simulink model "SVC_Modell_Changed"  (R2021a)
settings: Solver=ode1  StartTime=0.0  StopTime=t_Stop  FixedStep=0.1  RelTol=1e-3
values from neighbouring files (symbols this model uses):
  b_h = 0.5    [ParamterKamijiSVC_Changed.m]
  K_a = 0.1    [ParamterKamijiSVC_Changed.m]
  K_ac = 1.2    [ParamterKamijiSVC_Changed.m]
  K_vc = 6    [ParamterKamijiSVC_Changed.m]
  K_w = 0.9    [ParamterKamijiSVC_Changed.m]
  K_wc = 4    [ParamterKamijiSVC_Changed.m]
  n_h = 2    [ParamterKamijiSVC_Changed.m]
  P_kin = 1    [ParamterKamijiSVC_Changed.m]
  tau_a = 190    [ParamterKamijiSVC_Changed.m]
  tau_d = 7    [ParamterKamijiSVC_Changed.m]
  tau_LP = 0.1    [ParamterKamijiSVC_Changed.m]
undefined symbols (not defined in the file or in its folder): tau_MSI_unique
libraries: vrlib x3
settings Model: PauseTimes=1  Creator=BattiPerdator  LastModifiedBy=BattiPerdator

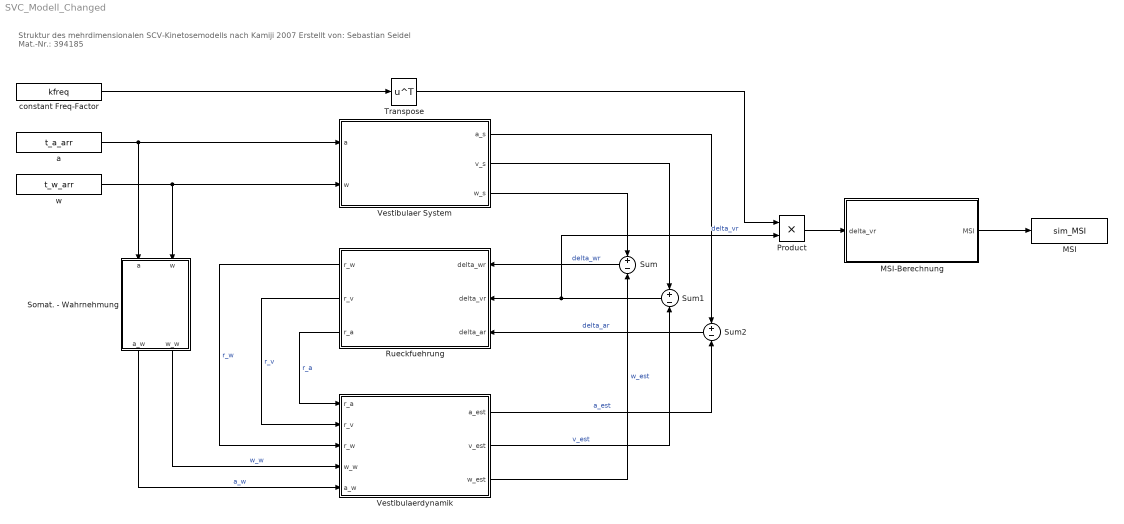
== system SVC_Modell_Changed ==
  note: Struktur des mehrdimensionalen SCV-Kinetosemodells nach Kamiji 2007
      | Erstellt von: Sebastian Seidel
      | Mat.-Nr.: 394185
  MSI : ToWorkspace  VariableName=sim_MSI  SampleTime=-1
  MSI-Berechnung : Subsystem
  Product : Product
  Rueckfuehrung : Subsystem
  Somat. - Wahrnehmung : Subsystem
  Sum : Sum  Inputs=+|-
  Sum1 : Sum  Inputs=+|-
  Sum2 : Sum  Inputs=+|-
  Transpose : Math  Operator=transpose  SaturateOnIntegerOverflow=on
  Vestibulaer System : Subsystem
  Vestibulaerdynamik : Subsystem
  "a " : FromWorkspace  VariableName=t_a_arr
  constant Freq-Factor : FromWorkspace  VariableName=kfreq
  w : FromWorkspace  VariableName=t_w_arr
  wires:
  w/1 -> Somat. - Wahrnehmung/2(w), Vestibulaer System/2(w)
  Somat. - Wahrnehmung/2(w_w) -> Vestibulaerdynamik/4(w_w)  "w_w"
  Somat. - Wahrnehmung/1(a_w) -> Vestibulaerdynamik/5(a_w)  "a_w"
  Vestibulaer System/1(a_s) -> Sum2/1
  Vestibulaer System/2(v_s) -> Sum1/1
  Vestibulaer System/3(w_s) -> Sum/1
  Vestibulaerdynamik/2(v_est) -> Sum1/2  "v_est"
  Rueckfuehrung/3(r_a) -> Vestibulaerdynamik/1(r_a)  "r_a"
  Rueckfuehrung/2(r_v) -> Vestibulaerdynamik/2(r_v)  "r_v"
  Rueckfuehrung/1(r_w) -> Vestibulaerdynamik/3(r_w)  "r_w"
  MSI-Berechnung/1(MSI) -> MSI/1
  Vestibulaerdynamik/1(a_est) -> Sum2/2  "a_est"
  Vestibulaerdynamik/3(w_est) -> Sum/2  "w_est"
  "a "/1 -> Somat. - Wahrnehmung/1(a), Vestibulaer System/1(a)
  Sum/1 -> Rueckfuehrung/1(delta_wr)  "delta_wr"
  Sum1/1 -> Product/2, Rueckfuehrung/2(delta_vr)  "delta_vr"
  Sum2/1 -> Rueckfuehrung/3(delta_ar)  "delta_ar"
  Product/1 -> MSI-Berechnung/1(delta_vr)
  constant Freq-Factor/1 -> Transpose/1
  Transpose/1 -> Product/1

== system SVC_Modell_Changed/MSI-Berechnung ==
  note: 0 ≤ MSI ≤ 1
  note: [-]
  note: [m/s²]
  delta_vr : Inport
  Hillfunktion : Subsystem
  Uebertragungsfunktion MSI : Subsystem
  MSI : Outport
  wires:
  delta_vr/1 -> Hillfunktion/1(delta_vr)
  Uebertragungsfunktion MSI/1(MSI) -> MSI/1
  Hillfunktion/1(h(delta_vr)) -> Uebertragungsfunktion MSI/1(h(delta_vr))

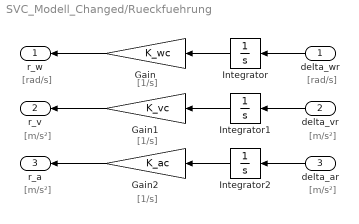
== system SVC_Modell_Changed/Rueckfuehrung ==
  note: [1/s]
  note: [rad/s]
  note: [m/s²]
  note: [m/s²]
  note: [rad/s]
  note: [m/s²]
  note: [m/s²]
  note: [1/s]
  note: [1/s]
  delta_wr : Inport
  delta_vr : Inport  Port=2
  delta_ar : Inport  Port=3
  Gain : Gain  Gain=K_wc
  Gain1 : Gain  Gain=K_vc
  Gain2 : Gain  Gain=K_ac
  Integrator : Integrator
  Integrator1 : Integrator
  Integrator2 : Integrator
  r_w : Outport
  r_v : Outport  Port=2
  r_a : Outport  Port=3
  wires:
  Gain/1 -> r_w/1
  Gain1/1 -> r_v/1
  Gain2/1 -> r_a/1
  delta_wr/1 -> Integrator/1
  Integrator/1 -> Gain/1
  delta_vr/1 -> Integrator1/1
  Integrator1/1 -> Gain1/1
  delta_ar/1 -> Integrator2/1
  Integrator2/1 -> Gain2/1

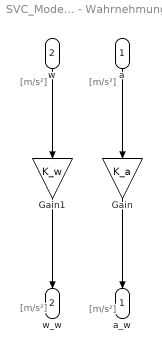
== system SVC_Modell_Changed/Somat. - Wahrnehmung ==
  note: [m/s²]
  note: [m/s²]
  note: [m/s²]
  note: [m/s²]
  a : Inport
  w : Inport  Port=2
  Gain : Gain  Gain=K_a
  Gain1 : Gain  Gain=K_w
  a_w : Outport
  w_w : Outport  Port=2
  wires:
  a/1 -> Gain/1
  Gain/1 -> a_w/1
  w/1 -> Gain1/1
  Gain1/1 -> w_w/1

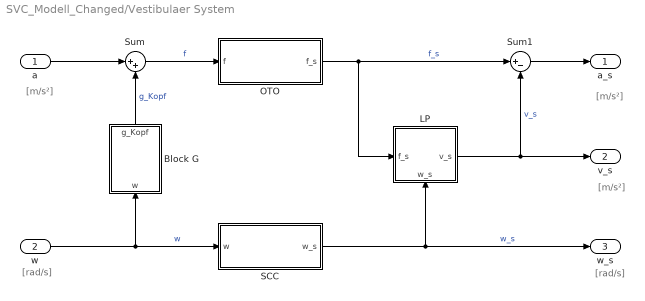
== system SVC_Modell_Changed/Vestibulaer System ==
  note: [m/s²]
  note: [m/s²]
  note: [m/s²]
  note: [rad/s]
  note: [rad/s]
  a : Inport
  w : Inport  Port=2
  Block G : Subsystem
  LP : Subsystem
      settings: PortSchema="{\"entries\":[{\"content\":{\"sides\":[{\"content\":{\"connectorIds\":[\"In1\"]},\"type\":\"ConnectorPlacement.EquallySpacedRectSide\",\"uuid\":\"fff2062c-4976-4e3f-90bd-2690d3961207\"},{\"content\":{\"connectorIds\":[\"Out1\"],\"side\":\"RIGHT\"},\"type\":\"ConnectorPlacement.EquallySpacedRectSide\",\"uuid\":\"f381f760-d607-432e-947a-7c2ed5cb0343\"},{\"content\":{\"connectorIds\":[],\"side\":\"TOP\"},\"type\":\"ConnectorPlacement.EquallySpacedRectSide\",\"uuid\":\"39b8ee05-57d9-4c64-9465-c67dc6896307\"},{\"content\":{\"connectorIds\":[\"In2\"],\"side\":\"BOTTOM\"},\"type\":\"ConnectorPlacement.EquallySpacedRectSide\",\"uuid\":\"95c95475-e280-41e4-b9b1-4b16bc0b77a9\"}]},\"type\":\"ConnectorPlacement.EquallySpacedConnector\",\"uuid\":\"1ef14ed4-54ab-4761-aaa8-a6dbdea02457\"}],\"packageUris\":[\"http://schema.mathworks.com/mf0/Connector/R2020b\"],\"version\":\"1.0\"}"
  OTO : Subsystem
  SCC : Subsystem
  Sum : Sum  Inputs=|++
  Sum1 : Sum  Inputs=|+-
  a_s : Outport
  v_s : Outport  Port=2
  w_s : Outport  Port=3
  wires:
  Block G/1(g_Kopf) -> Sum/2  "g_Kopf"
  a/1 -> Sum/1
  Sum/1 -> OTO/1(f)  "f"
  Sum1/1 -> a_s/1
  OTO/1(f_s) -> LP/1(f_s), Sum1/1  "f_s"
  LP/1(v_s) -> Sum1/2, v_s/1  "v_s"
  w/1 -> SCC/1(w), Block G/1(w)  "w"
  SCC/1(w_s) -> LP/2(w_s), w_s/1  "w_s"

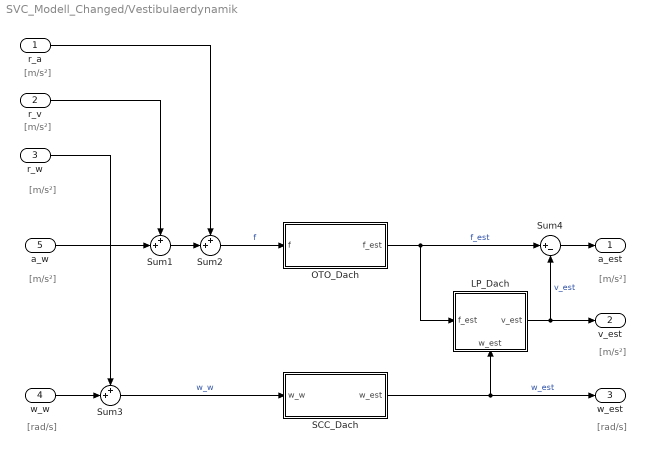
== system SVC_Modell_Changed/Vestibulaerdynamik ==
  note: [m/s²]
  note: [m/s²]
  note: [m/s²]
  note: [m/s²]
  note: [m/s²]
  note: [m/s²]
  note: [rad/s]
  note: [rad/s]
  r_a : Inport
  r_v : Inport  Port=2
  r_w : Inport  Port=3
  w_w : Inport  Port=4
  a_w : Inport  Port=5
  LP_Dach : Subsystem
      settings: PortSchema="{\"entries\":[{\"content\":{\"sides\":[{\"content\":{\"connectorIds\":[\"In1\"]},\"type\":\"ConnectorPlacement.EquallySpacedRectSide\",\"uuid\":\"4576b9b0-b7f1-41f5-8e73-fb131cbc4e5d\"},{\"content\":{\"connectorIds\":[\"Out1\"],\"side\":\"RIGHT\"},\"type\":\"ConnectorPlacement.EquallySpacedRectSide\",\"uuid\":\"977d9525-9a1c-46d7-8515-3c5f667f8023\"},{\"content\":{\"connectorIds\":[],\"side\":\"TOP\"},\"type\":\"ConnectorPlacement.EquallySpacedRectSide\",\"uuid\":\"54849022-6004-4c1b-9656-1ca460f60ce4\"},{\"content\":{\"connectorIds\":[\"In2\"],\"side\":\"BOTTOM\"},\"type\":\"ConnectorPlacement.EquallySpacedRectSide\",\"uuid\":\"a9bd4e87-4f64-4d0a-b6c8-09ec812a1771\"}]},\"type\":\"ConnectorPlacement.EquallySpacedConnector\",\"uuid\":\"028b9623-ac93-41b0-b7c2-ce6b7edafabd\"}],\"packageUris\":[\"http://schema.mathworks.com/mf0/Connector/R2020b\"],\"version\":\"1.0\"}"
  OTO_Dach : Subsystem
  SCC_Dach : Subsystem
  Sum1 : Sum  Inputs=++|
  Sum2 : Sum  Inputs=++|
  Sum3 : Sum  Inputs=++|
  Sum4 : Sum  Inputs=|+-
  a_est : Outport
  v_est : Outport  Port=2
  w_est : Outport  Port=3
  wires:
  Sum1/1 -> Sum2/2
  r_v/1 -> Sum1/1
  a_w/1 -> Sum1/2
  w_w/1 -> Sum3/2
  r_w/1 -> Sum3/1
  r_a/1 -> Sum2/1
  Sum2/1 -> OTO_Dach/1(f)  "f"
  Sum4/1 -> a_est/1
  OTO_Dach/1(f_est) -> LP_Dach/1(f_est), Sum4/1  "f_est"
  Sum3/1 -> SCC_Dach/1(w_w)  "w_w"
  SCC_Dach/1(w_est) -> LP_Dach/2(w_est), w_est/1  "w_est"
  LP_Dach/1(v_est) -> Sum4/2, v_est/1  "v_est"

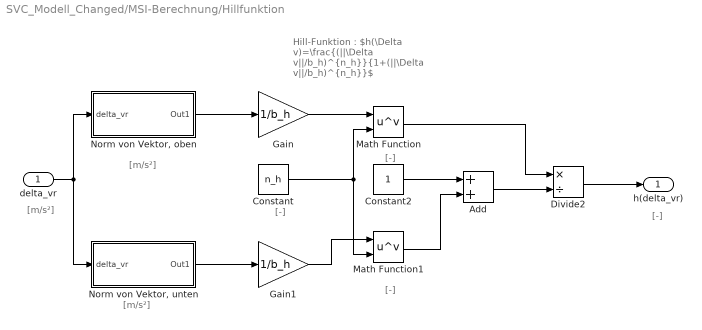
== system SVC_Modell_Changed/MSI-Berechnung/Hillfunktion ==
  note: Hill-Funktion :
      | $h(\Delta v)=\frac{(||\Delta v||/b_h)^{n_h}}{1+(||\Delta v||/b_h)^{n_h}}$
  note: [-]
  note: [-]
  note: [-]
  note: [m/s²]
  note: [m/s²]
  note: [m/s²]
  note: [-]
  delta_vr : Inport
  Add : Sum
  Constant : Constant  Value=n_h
  Constant2 : Constant
  Divide2 : Product  Inputs=*/
  Gain : Gain  Gain=1/b_h
  Gain1 : Gain  Gain=1/b_h
  Math Function : Math  Operator=pow  SaturateOnIntegerOverflow=on
  Math Function1 : Math  Operator=pow  SaturateOnIntegerOverflow=on
  "Norm von Vektor, oben" : Subsystem
  "Norm von Vektor, unten" : Subsystem
  h(delta_vr) : Outport
  wires:
  Constant2/1 -> Add/1
  Math Function1/1 -> Add/2
  Divide2/1 -> h(delta_vr)/1
  Add/1 -> Divide2/2
  Math Function/1 -> Divide2/1
  delta_vr/1 -> "Norm von Vektor, unten"/1(delta_vr), "Norm von Vektor, oben"/1(delta_vr)
  Constant/1 -> Math Function1/2, Math Function/2
  "Norm von Vektor, oben"/1(Out1) -> Gain/1
  Gain/1 -> Math Function/1
  "Norm von Vektor, unten"/1(Out1) -> Gain1/1
  Gain1/1 -> Math Function1/1

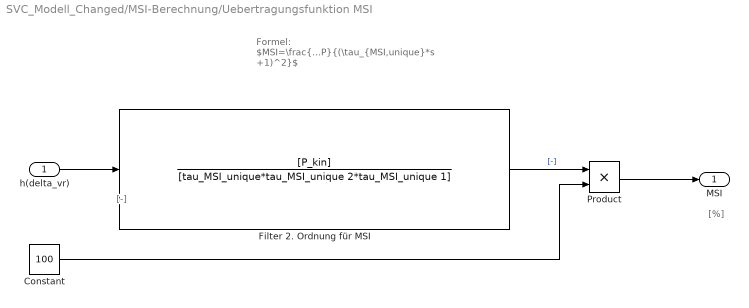
== system SVC_Modell_Changed/MSI-Berechnung/Uebertragungsfunktion MSI ==
  note: Formel:
      | $MSI=\frac{P}{(\tau_{MSI,unique}*s +1)^2}$
  note: [%]
  note: [-]
  h(delta_vr) : Inport
  Constant : Constant  Value=100
  Filter 2. Ordnung für MSI : TransferFcn  Numerator=[P_kin]  Denominator=[tau_MSI_unique*tau_MSI_unique 2*tau_MSI_unique 1]  ParameterTunability=Optimized
  Product : Product
  MSI : Outport
  wires:
  h(delta_vr)/1 -> Filter 2. Ordnung für MSI/1
  Product/1 -> MSI/1
  Filter 2. Ordnung für MSI/1 -> Product/1  "[-]"
  Constant/1 -> Product/2

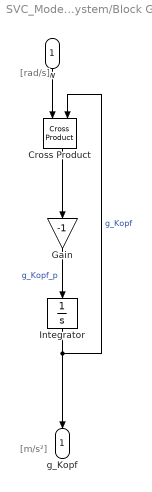
== system SVC_Modell_Changed/Vestibulaer System/Block G ==
  note: [m/s²]
  note: [rad/s]
  w : Inport
  Cross Product : vrlib/Utilities/Cross Product
  Gain : Gain  Gain=-1
  Integrator : Integrator
  g_Kopf : Outport
  wires:
  Cross Product/1 -> Gain/1
  Gain/1 -> Integrator/1  "g_Kopf_p"
  Integrator/1 -> Cross Product/2, g_Kopf/1  "g_Kopf"
  w/1 -> Cross Product/1

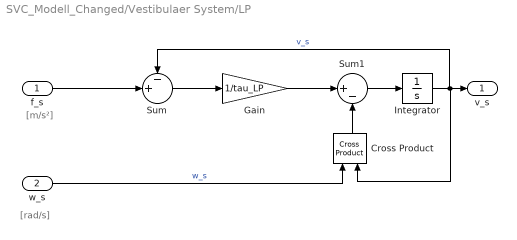
== system SVC_Modell_Changed/Vestibulaer System/LP ==
  note: [m/s²]
  note: [rad/s]
  f_s : Inport
  w_s : Inport  Port=2
  Cross Product : vrlib/Utilities/Cross Product
  Gain : Gain  Gain=1/tau_LP
  Integrator : Integrator
  Sum : Sum  Inputs=-+|
  Sum1 : Sum  Inputs=|+-
  v_s : Outport
  wires:
  f_s/1 -> Sum/2
  Sum/1 -> Gain/1
  Gain/1 -> Sum1/1
  Sum1/1 -> Integrator/1
  Integrator/1 -> Cross Product/2, v_s/1, Sum/1  "v_s"
  Cross Product/1 -> Sum1/2
  w_s/1 -> Cross Product/1  "w_s"

== system SVC_Modell_Changed/Vestibulaer System/OTO ==
  note: [m/s²]
  note: [m/s²]
  f : Inport
  f_s : Outport
  wires:
  f/1 -> f_s/1

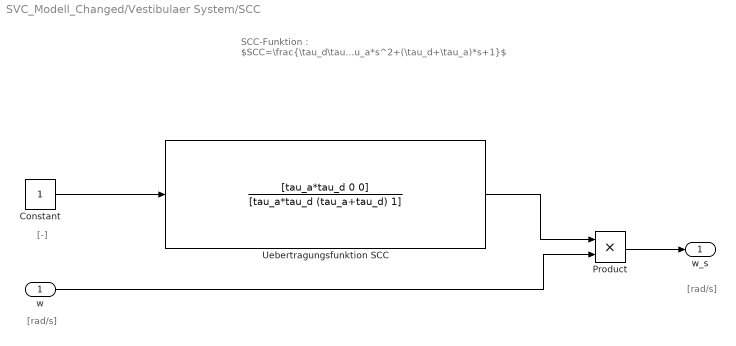
== system SVC_Modell_Changed/Vestibulaer System/SCC ==
  note: [-]
  note: [rad/s]
  note: [rad/s]
  note: SCC-Funktion :
      | $SCC=\frac{\tau_d\tau_a*s}{\tau_d\tau_a*s^2+(\tau_d+\tau_a)*s+1}$
  w : Inport
  Constant : Constant
  Product : Product
  Uebertragungsfunktion SCC : TransferFcn  Numerator=[tau_a*tau_d 0 0]  Denominator=[tau_a*tau_d (tau_a+tau_d) 1]
  w_s : Outport
  wires:
  Product/1 -> w_s/1
  w/1 -> Product/2
  Uebertragungsfunktion SCC/1 -> Product/1
  Constant/1 -> Uebertragungsfunktion SCC/1

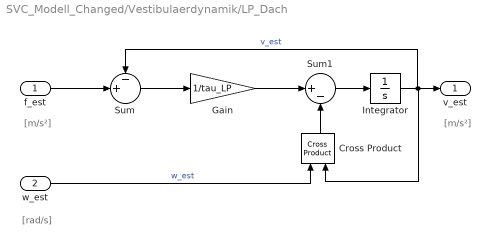
== system SVC_Modell_Changed/Vestibulaerdynamik/LP_Dach ==
  note: [m/s²]
  note: [m/s²]
  note: [rad/s]
  f_est : Inport
  w_est : Inport  Port=2
  Cross Product : vrlib/Utilities/Cross Product
  Gain : Gain  Gain=1/tau_LP
  Integrator : Integrator
  Sum : Sum  Inputs=-+|
  Sum1 : Sum  Inputs=|+-
  v_est : Outport
  wires:
  Sum1/1 -> Integrator/1
  Cross Product/1 -> Sum1/2
  Integrator/1 -> v_est/1, Cross Product/2, Sum/1  "v_est"
  Sum/1 -> Gain/1
  Gain/1 -> Sum1/1
  f_est/1 -> Sum/2
  w_est/1 -> Cross Product/1  "w_est"

== system SVC_Modell_Changed/Vestibulaerdynamik/OTO_Dach ==
  note: [m/s²]
  note: [m/s²]
  f : Inport
  f_est : Outport
  wires:
  f/1 -> f_est/1

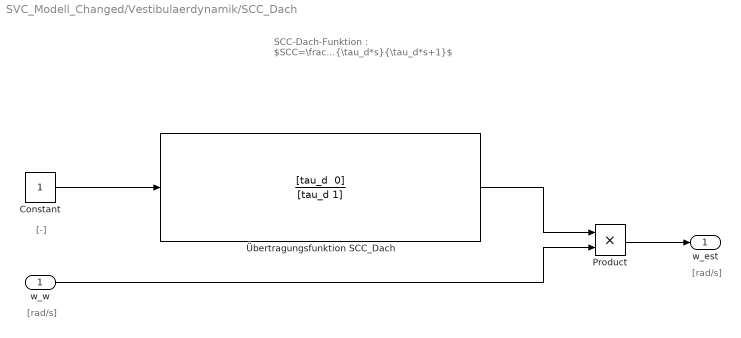
== system SVC_Modell_Changed/Vestibulaerdynamik/SCC_Dach ==
  note: [-]
  note: [rad/s]
  note: [rad/s]
  note: SCC-Dach-Funktion :
      | $SCC=\frac{\tau_d*s}{\tau_d*s+1}$
  w_w : Inport
  Constant : Constant
  Product : Product
  Übertragungsfunktion SCC_Dach : TransferFcn  Numerator="[tau_d  0]"  Denominator=[tau_d 1]
  w_est : Outport
  wires:
  Product/1 -> w_est/1
  w_w/1 -> Product/2
  Constant/1 -> Übertragungsfunktion SCC_Dach/1
  Übertragungsfunktion SCC_Dach/1 -> Product/1

== system SVC_Modell_Changed/MSI-Berechnung/Hillfunktion/Norm von Vektor, oben ==
  delta_vr : Inport
  Dot Product : DotProduct  InputSameDT=on  OutDataTypeStr=Inherit: Inherit via internal rule
  Sqrt : Sqrt  SaturateOnIntegerOverflow=on
  Out1 : Outport
  wires:
  Dot Product/1 -> Sqrt/1
  Sqrt/1 -> Out1/1
  delta_vr/1 -> Dot Product/1, Dot Product/2

== system SVC_Modell_Changed/MSI-Berechnung/Hillfunktion/Norm von Vektor, unten ==
  delta_vr : Inport
  Dot Product : DotProduct  InputSameDT=on  OutDataTypeStr=Inherit: Inherit via internal rule
  Sqrt : Sqrt  SaturateOnIntegerOverflow=on
  Out1 : Outport
  wires:
  Dot Product/1 -> Sqrt/1
  Sqrt/1 -> Out1/1
  delta_vr/1 -> Dot Product/1, Dot Product/2
